simulink model "W02_2_goto_offline"  (R2024b)
settings: Solver=FixedStepDiscrete  StartTime=0.0  StopTime=T_end  FixedStep=Ts  RelTol=1e-3
values from neighbouring files (symbols this model uses):
  animate = 1    [W02_setup.m]
  Kpsi = 4.0    (= 4)    [W02_setup.m]
  Kv = 1.0    (= 1)    [W02_setup.m]
  theta_goal = deg2rad(145)    [W02_setup.m]
  tol_d = 0.05    [W02_setup.m]
  tol_th = deg2rad(1.0)    [W02_setup.m]
  Ts = 0.05    [W02_setup.m]
  v_max = 2.0    (= 2)    [W02_setup.m]
  w_max = 2.0    (= 2)    [W02_setup.m]
  x0 = [5.544445; 5.544445; 0]    [W02_setup.m]    (also in tidy_layout.m = min(P(:,1)))
  x_goal = 5.0    (= 5)    [W02_setup.m]
  y_goal = 5.0    (= 5)    [W02_setup.m]
settings Model: Creator=admin  LastModifiedBy=admin

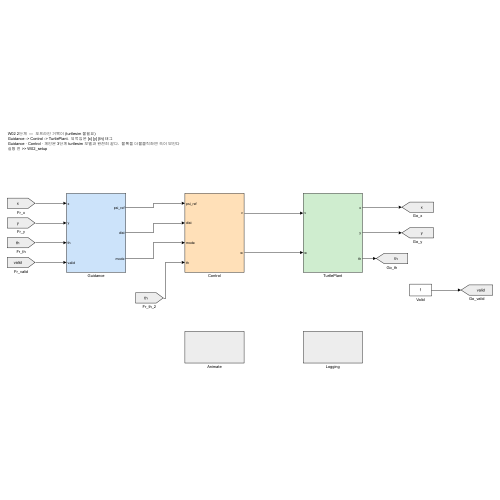
[thumbnail: Simulink's stored preview of the top-level diagram]
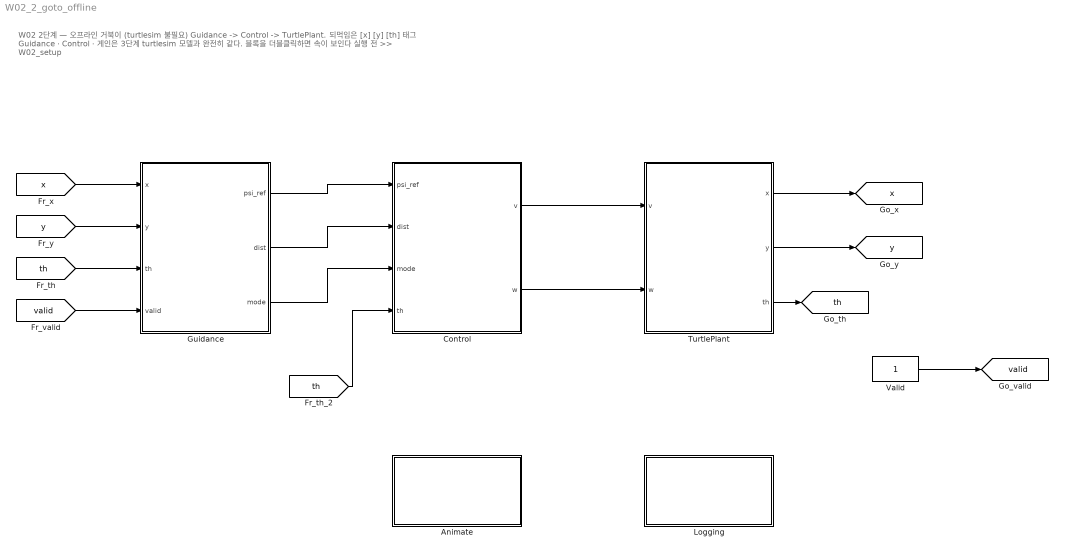
== system W02_2_goto_offline ==
  note: W02 2단계  —  오프라인 거북이 (turtlesim 불필요)
      | Guidance -> Control -> TurtlePlant.  되먹임은 [x] [y] [th] 태그
      | Guidance · Control · 게인은 3단계 turtlesim 모델과 완전히 같다.  블록을 더블클릭하면 속이 보인다
      | 실행 전 >> W02_setup
  Animate : Subsystem
  Control : Subsystem
  Guidance : Subsystem
  Logging : Subsystem
  TurtlePlant : Subsystem
  Valid : Constant
  tag scope: th=global, valid=global, x=global, y=global
  wires:
  [x] -> Guidance/1(x)
  [y] -> Guidance/2(y)
  [th] -> Guidance/3(th)
  [valid] -> Guidance/4(valid)
  Guidance/1(psi_ref) -> Control/1(psi_ref)
  Guidance/2(dist) -> Control/2(dist)
  Guidance/3(mode) -> Control/3(mode)
  Control/1(v) -> TurtlePlant/1(v)
  Control/2(w) -> TurtlePlant/2(w)
  TurtlePlant/1(x) -> [x]
  TurtlePlant/2(y) -> [y]
  Valid/1 -> [valid]
  TurtlePlant/3(th) -> [th]
  [th] -> Control/4(th)

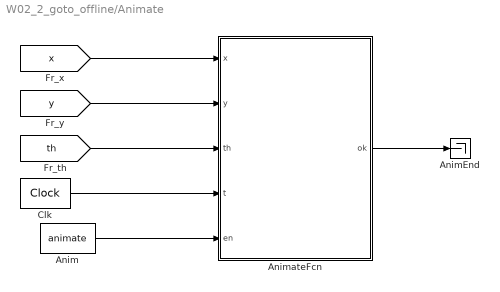
== system W02_2_goto_offline/Animate ==
  Anim : Constant  Value=animate
  AnimEnd : Terminator
  AnimateFcn : MATLAB Function  TreatAsAtomicUnit=on
  Clk : DigitalClock  SampleTime=Ts
  wires:
  [x] -> AnimateFcn/1(x)
  [y] -> AnimateFcn/2(y)
  [th] -> AnimateFcn/3(th)
  Clk/1 -> AnimateFcn/4(t)
  Anim/1 -> AnimateFcn/5(en)
  AnimateFcn/1(ok) -> AnimEnd/1

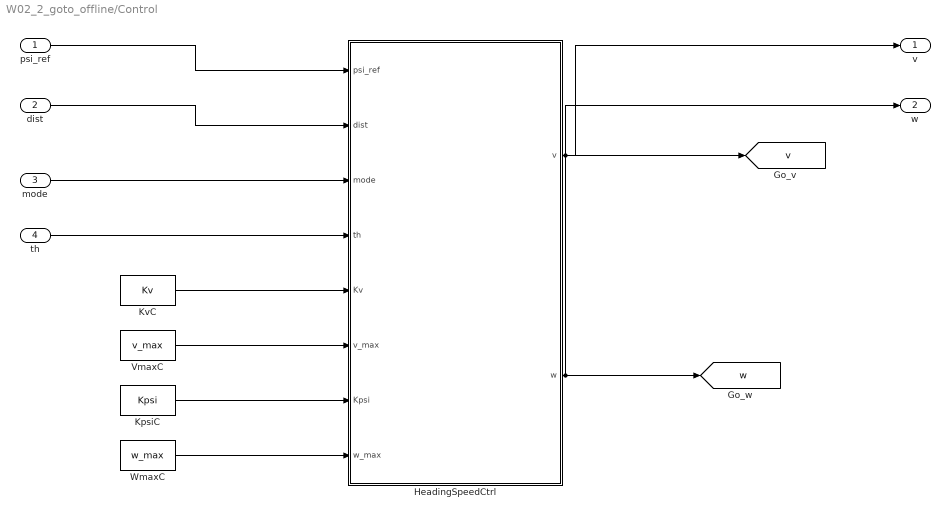
== system W02_2_goto_offline/Control ==
  psi_ref : Inport
  dist : Inport  Port=2
  mode : Inport  Port=3
  th : Inport  Port=4
  HeadingSpeedCtrl : MATLAB Function  TreatAsAtomicUnit=on
  KpsiC : Constant  Value=Kpsi
  KvC : Constant  Value=Kv
  VmaxC : Constant  Value=v_max
  WmaxC : Constant  Value=w_max
  v : Outport
  w : Outport  Port=2
  tag scope: v=global, w=global
  wires:
  psi_ref/1 -> HeadingSpeedCtrl/1(psi_ref)
  dist/1 -> HeadingSpeedCtrl/2(dist)
  mode/1 -> HeadingSpeedCtrl/3(mode)
  th/1 -> HeadingSpeedCtrl/4(th)
  KvC/1 -> HeadingSpeedCtrl/5(Kv)
  VmaxC/1 -> HeadingSpeedCtrl/6(v_max)
  KpsiC/1 -> HeadingSpeedCtrl/7(Kpsi)
  WmaxC/1 -> HeadingSpeedCtrl/8(w_max)
  HeadingSpeedCtrl/2(w) -> [w], w/1
  HeadingSpeedCtrl/1(v) -> [v], v/1

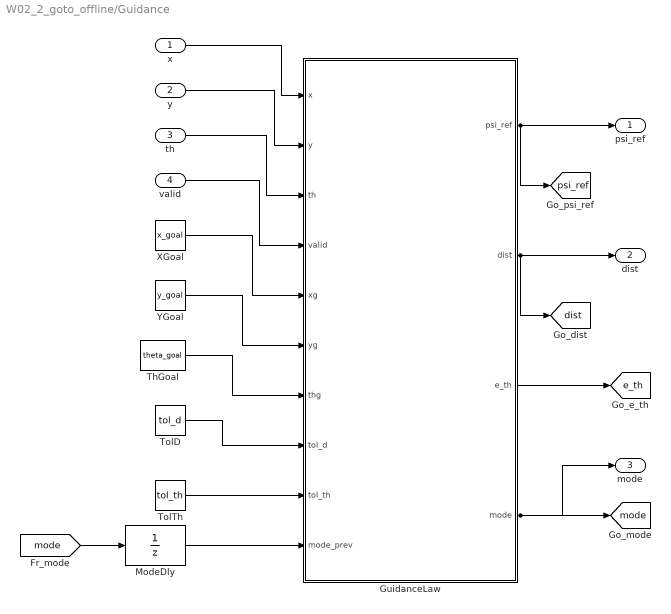
== system W02_2_goto_offline/Guidance ==
  x : Inport
  y : Inport  Port=2
  th : Inport  Port=3
  valid : Inport  Port=4
  GuidanceLaw : MATLAB Function  TreatAsAtomicUnit=on
  ModeDly : UnitDelay  InitialCondition=1  SampleTime=Ts  HasFrameUpgradeWarning=on
  ThGoal : Constant  Value=theta_goal
  TolD : Constant  Value=tol_d
  TolTh : Constant  Value=tol_th
  XGoal : Constant  Value=x_goal
  YGoal : Constant  Value=y_goal
  psi_ref : Outport
  dist : Outport  Port=2
  mode : Outport  Port=3
  tag scope: dist=global, e_th=global, mode=global, psi_ref=global
  wires:
  y/1 -> GuidanceLaw/2(y)
  x/1 -> GuidanceLaw/1(x)
  valid/1 -> GuidanceLaw/4(valid)
  th/1 -> GuidanceLaw/3(th)
  XGoal/1 -> GuidanceLaw/5(xg)
  TolTh/1 -> GuidanceLaw/9(tol_th)
  YGoal/1 -> GuidanceLaw/6(yg)
  TolD/1 -> GuidanceLaw/8(tol_d)
  ThGoal/1 -> GuidanceLaw/7(thg)
  ModeDly/1 -> GuidanceLaw/10(mode_prev)
  GuidanceLaw/1(psi_ref) -> psi_ref/1, [psi_ref]
  GuidanceLaw/2(dist) -> dist/1, [dist]
  GuidanceLaw/3(e_th) -> [e_th]
  GuidanceLaw/4(mode) -> mode/1, [mode]
  [mode] -> ModeDly/1

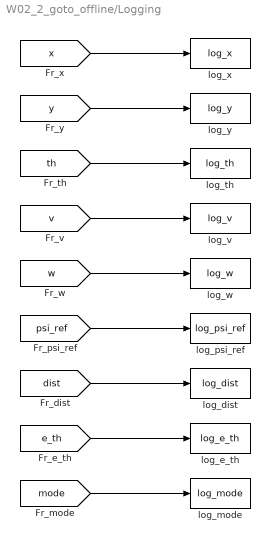
== system W02_2_goto_offline/Logging ==
  log_dist : ToWorkspace  VariableName=log_dist  SaveFormat=Timeseries  SampleTime=Ts
  log_e_th : ToWorkspace  VariableName=log_e_th  SaveFormat=Timeseries  SampleTime=Ts
  log_mode : ToWorkspace  VariableName=log_mode  SaveFormat=Timeseries  SampleTime=Ts
  log_psi_ref : ToWorkspace  VariableName=log_psi_ref  SaveFormat=Timeseries  SampleTime=Ts
  log_th : ToWorkspace  VariableName=log_th  SaveFormat=Timeseries  SampleTime=Ts
  log_v : ToWorkspace  VariableName=log_v  SaveFormat=Timeseries  SampleTime=Ts
  log_w : ToWorkspace  VariableName=log_w  SaveFormat=Timeseries  SampleTime=Ts
  log_x : ToWorkspace  VariableName=log_x  SaveFormat=Timeseries  SampleTime=Ts
  log_y : ToWorkspace  VariableName=log_y  SaveFormat=Timeseries  SampleTime=Ts
  wires:
  [x] -> log_x/1
  [y] -> log_y/1
  [th] -> log_th/1
  [v] -> log_v/1
  [w] -> log_w/1
  [psi_ref] -> log_psi_ref/1
  [dist] -> log_dist/1
  [e_th] -> log_e_th/1
  [mode] -> log_mode/1

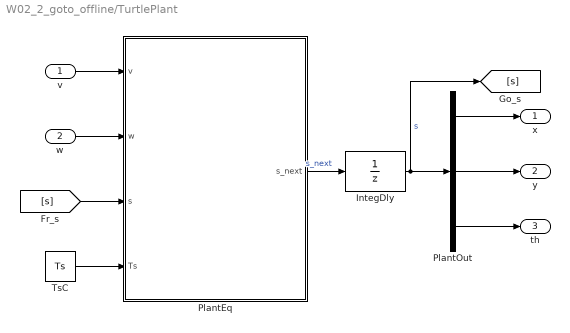
== system W02_2_goto_offline/TurtlePlant ==
  v : Inport
  w : Inport  Port=2
  IntegDly : UnitDelay  InitialCondition=x0  SampleTime=Ts  HasFrameUpgradeWarning=on
  PlantEq : MATLAB Function  TreatAsAtomicUnit=on
  PlantOut : Demux  Outputs=3
  TsC : Constant  Value=Ts
  x : Outport
  y : Outport  Port=2
  th : Outport  Port=3
  wires:
  v/1 -> PlantEq/1(v)
  IntegDly/1 -> PlantOut/1, [s]  "s"
  w/1 -> PlantEq/2(w)
  PlantOut/3 -> th/1
  PlantOut/2 -> y/1
  PlantOut/1 -> x/1
  TsC/1 -> PlantEq/4(Ts)
  PlantEq/1(s_next) -> IntegDly/1  "s_next"
  [s] -> PlantEq/3(s)

== matlab function W02_2_goto_offline/Control/HeadingSpeedCtrl ==
  data: psi_ref input; v output; dist input; mode input; th input; Kv input; v_max input; Kpsi input; w_max input; w output
function [v, w] = HeadingSpeedCtrl(psi_ref, dist, mode, th, Kv, v_max, Kpsi, w_max)
%#codegen
% Heading control (P) and speed control (P on distance).
% turtlesim is kinematic: cmd_vel sets the velocity directly,
% so no yaw-rate (D) term or thrust model is needed here.

e = mod(psi_ref - th + pi, 2*pi) - pi;     % heading error, [-pi, pi)
w = min(max(Kpsi*e, -w_max), w_max);

if mode == 1
    % slow down near the goal; do not drive while facing away from it
    v = min(Kv*dist, v_max) * max(cos(e), 0);
elseif mode == 2
    v = 0;                                  % turn on the spot
else
    v = 0;  w = 0;                          % done
end

== matlab function W02_2_goto_offline/Guidance/GuidanceLaw ==
  data: x input; psi_ref output; y input; th input; valid input; xg input; yg input; thg input; tol_d input; tol_th input; mode_prev input; dist output; e_th output; mode output
function [psi_ref, dist, e_th, mode] = GuidanceLaw(x, y, th, valid, xg, yg, thg, tol_d, tol_th, mode_prev)
%#codegen
% Go-to-pose guidance for turtlesim. One thing at a time:
%   mode 1 GO    : head for the goal point.   dist < tol_d   -> mode 2
%   mode 2 ALIGN : turn to the goal heading.  |e_th| < tol_th -> mode 3
%   mode 3 DONE  : stay still.  goal moved away (dist > 3*tol_d) -> mode 1
% turtlesim frame: x right, y up, theta counter-clockwise from +x.

dist = sqrt((xg - x)^2 + (yg - y)^2);
mode = mode_prev;

if valid < 0.5              % no pose received yet -> do not move
    psi_ref = th; e_th = 0; mode = 1;
    return
end

if mode == 1
    if dist < tol_d, mode = 2; end
elseif mode == 2
    if dist > 3*tol_d
        mode = 1;
    elseif abs(ssa(thg - th)) < tol_th
        mode = 3;
    end
else
    if dist > 3*tol_d, mode = 1; end
end

if mode == 1
    psi_ref = atan2(yg - y, xg - x);   % bearing to the goal point
else
    psi_ref = thg;                     % final heading
end
e_th = ssa(thg - th);                  % final-heading error (for logging)
end

function a = ssa(a)
% smallest signed angle, [-pi, pi)
a = mod(a + pi, 2*pi) - pi;
end

== matlab function W02_2_goto_offline/TurtlePlant/PlantEq ==
  data: v input; s_next output; w input; s input; Ts input
function s_next = PlantEq(v, w, s, Ts)
%#codegen
% Same kinematics as turtlesim_node (turtle.cpp):
%   theta += w*dt,  x += v*cos(theta)*dt,  y += v*sin(theta)*dt
% The turtle stops at the walls (0 .. 11.0889).
x = s(1);  y = s(2);  th = s(3);
th = th + w*Ts;
th = mod(th + pi, 2*pi) - pi;
x  = x + v*cos(th)*Ts;
y  = y + v*sin(th)*Ts;
x  = min(max(x, 0), 11.088889);
y  = min(max(y, 0), 11.088889);
s_next = [x; y; th];

== matlab function W02_2_goto_offline/Animate/AnimateFcn ==
  data: x input; ok output; y input; th input; t input; en input
function ok = AnimateFcn(x, y, th, t, en)
%#codegen
% Live plot of the hull. Plotting is plain MATLAB, so it is
% declared extrinsic.
coder.extrinsic('W02_animate');
ok = 1;
if en > 0.5
    W02_animate(x, y, th, t);
end
